simulink model "W06_city_highway_cs"  (R2019a)
settings: Solver=ode5  StartTime=0.0  StopTime=inf  FixedStep=1/60  RelTol=1e-3
PreLoadFcn:
  | mbxruntime.callbacks.PreLoadFcn(bdroot);
PostLoadFcn:
  | mbxruntime.callbacks.PostLoadFcn(bdroot);
InitFcn:
  | mbxruntime.callbacks.InitFcn(bdroot);
StartFcn:
  | mbxruntime.callbacks.StartFcn(bdroot);
StopFcn:
  | mbxruntime.callbacks.StopFcn(bdroot);
model workspace: external: MAT-File .\W06_city_highway_cs_hws.mat (data not in the file)
undefined symbols (not defined in the file or in its folder): DiscIntNeverNeededParam, FovAzimuth, FovAzimuthDefined, FovElevation, FovElevationDefined, Header, InitImageOutputDir, LocationX, LocationXDefined, LocationY, LocationYDefined, LocationZ, LocationZDefined, Orientation, OrientationPitch, OrientationPitchDefined, OrientationRoll, OrientationRollDefined, OrientationYaw, OrientationYawDefined, Poses, Poses_SL_Info, Position, W06_city_highway_cs_0270c22595f3b0e3, W06_city_highway_cs_086892688dd32ddc, W06_city_highway_cs_328c49ac39fca66b, W06_city_highway_cs_35ce05381b8ebe8c, W06_city_highway_cs_47b384f162638175, W06_city_highway_cs_766f76ce4de94dd5, W06_city_highway_cs_8c547f67cb81ffba, W06_city_highway_cs_aed52f2a7724a4f9, W06_city_highway_cs_Audi_A8_Sedan_1_Path_pathUniqueID, W06_city_highway_cs_b74cbb1f9f7331b5, W06_city_highway_cs_Citroen_C3_Hatchback_1_Path_pathUniqueID, W06_city_highway_cs_d395f8835e0c28b3, W06_city_highway_cs_e5f9d1759e19e2b4, W06_city_highway_cs_Toyota_Previa_MPV_1_Path_pathUniqueID
libraries: adeye_lib x26, simulink_extras x24, robotlib x7, sharedtransform x4, PreScanSimulinkLibrary x2, PreScanUsefulBlocks x1
(part 5 of 8)

== system W06_city_highway_cs/BMW_X5_SUV_2/HumViewCamera_CM_Demux ==
  In1 : Inport
  Selector : Selector  NumberOfDimensions=2  InputPortWidth=3  IndexOptions=Index vector (dialog),Index vector (dialog)  Indices=-1,1:hres  OutputSizes=1,1
  Selector1 : Selector  NumberOfDimensions=2  InputPortWidth=3  IndexOptions=Index vector (dialog),Index vector (dialog)  Indices=-1,hres+1:hres*2  OutputSizes=1,1
  Selector2 : Selector  NumberOfDimensions=2  InputPortWidth=3  IndexOptions=Index vector (dialog),Index vector (dialog)  Indices=-1,hres*2+1:hres*3  OutputSizes=1,1
  R : Outport
  G : Outport  Port=2
  B : Outport  Port=3
  wires:
  In1/1 -> Selector1/1, Selector/1, Selector2/1
  Selector/1 -> R/1
  Selector1/1 -> G/1
  Selector2/1 -> B/1

== system W06_city_highway_cs/BMW_X5_SUV_2/Mux_Camera_1_TA ==
  Location : Inport  Tag=inport/Camera_TA  OutDataTypeStr=double  PortDimensions=3  BusOutputAsStruct=on
  Orientation : Inport  Tag=inport/Camera_TA  Port=2  OutDataTypeStr=double  PortDimensions=3  BusOutputAsStruct=on
  IntensityFactorRGBMono : Inport  Tag=inport/Camera_TA  Port=3  OutDataTypeStr=double  PortDimensions=3  BusOutputAsStruct=on
  FoVAzimuth : Inport  Tag=inport/Camera_TA  Port=4  OutDataTypeStr=double  PortDimensions=1  BusOutputAsStruct=on
  FoVElevation : Inport  Tag=inport/Camera_TA  Port=5  OutDataTypeStr=double  PortDimensions=1  BusOutputAsStruct=on
  MisAlignMountPos : Inport  Tag=inport/Camera_TA  Port=6  OutDataTypeStr=double  PortDimensions=3  BusOutputAsStruct=on
  MisAlignMountOrient : Inport  Tag=inport/Camera_TA  Port=7  OutDataTypeStr=double  PortDimensions=3  BusOutputAsStruct=on
  Bus Assignment TA : BusAssignment  AssignedSignals=LocationX,LocationY,LocationZ,OrientationRoll,OrientationPitch,OrientationYaw,IntensityFactorR,IntensityFactorG,IntensityFactorB,FoVAzimuth,FoVElevation,MisalignMountPosX,MisalignMountPosY,MisalignMountPosZ,MisalignMountOrientX,MisalignMountOrientY,MisalignMountOrientZ,LocationXDefined,LocationYDefined,LocationZDefined,OrientationRollDefined,OrientationPitchDefined,OrientationYawDefined,IntensityFactorRDefined,IntensityFactorGDefined,IntensityFactorBDefined,FoVAzimuthDefined,FoVElevationDefined,MisalignMountPosXDefined,MisalignMountPosYDefined,MisalignMountPosZDefined,MisalignMountOrientXDefined,MisalignMountOrientYDefined,MisalignMountOrientZDefined
  ENABLE : Constant  Tag=ENABLE  Value=true
  IntensityFactorRGBMono_vec : Demux  Outputs=3
  Location_vec : Demux  Outputs=3
  MisAlignMountOrient_vec : Demux  Outputs=3
  MisAlignMountPos_vec : Demux  Outputs=3
  Orientation_vec : Demux  Outputs=3
  TA_bus : Subsystem
  TA : Outport  Tag=outport/Camera_TA/CameraSensor  OutDataTypeStr=Bus: PRESCAN_CAMERASENSOR_TA  PortDimensions=1  SampleTime=1/60
  wires:
  Bus Assignment TA/1 -> TA/1
  Location/1 -> Location_vec/1
  Location_vec/1 -> Bus Assignment TA/2
  Location_vec/2 -> Bus Assignment TA/3
  Location_vec/3 -> Bus Assignment TA/4
  Orientation/1 -> Orientation_vec/1
  Orientation_vec/1 -> Bus Assignment TA/5
  Orientation_vec/2 -> Bus Assignment TA/6
  Orientation_vec/3 -> Bus Assignment TA/7
  IntensityFactorRGBMono/1 -> IntensityFactorRGBMono_vec/1
  IntensityFactorRGBMono_vec/1 -> Bus Assignment TA/8
  IntensityFactorRGBMono_vec/2 -> Bus Assignment TA/9
  IntensityFactorRGBMono_vec/3 -> Bus Assignment TA/10
  FoVAzimuth/1 -> Bus Assignment TA/11
  FoVElevation/1 -> Bus Assignment TA/12
  MisAlignMountPos/1 -> MisAlignMountPos_vec/1
  MisAlignMountPos_vec/1 -> Bus Assignment TA/13
  MisAlignMountPos_vec/2 -> Bus Assignment TA/14
  MisAlignMountPos_vec/3 -> Bus Assignment TA/15
  MisAlignMountOrient/1 -> MisAlignMountOrient_vec/1
  MisAlignMountOrient_vec/1 -> Bus Assignment TA/16
  MisAlignMountOrient_vec/2 -> Bus Assignment TA/17
  MisAlignMountOrient_vec/3 -> Bus Assignment TA/18
  ENABLE/1 -> Bus Assignment TA/19, Bus Assignment TA/20, Bus Assignment TA/21, Bus Assignment TA/22, Bus Assignment TA/23, Bus Assignment TA/24, Bus Assignment TA/25, Bus Assignment TA/26, Bus Assignment TA/27, Bus Assignment TA/28, Bus Assignment TA/29, Bus Assignment TA/30, Bus Assignment TA/31, Bus Assignment TA/32, Bus Assignment TA/33, Bus Assignment TA/34, Bus Assignment TA/35
  TA_bus/1(bus) -> Bus Assignment TA/1

== system W06_city_highway_cs/BMW_X5_SUV_2/Mux_Camera_2_TA ==
  Location : Inport  Tag=inport/Camera_TA  OutDataTypeStr=double  PortDimensions=3  BusOutputAsStruct=on
  Orientation : Inport  Tag=inport/Camera_TA  Port=2  OutDataTypeStr=double  PortDimensions=3  BusOutputAsStruct=on
  IntensityFactorRGBMono : Inport  Tag=inport/Camera_TA  Port=3  OutDataTypeStr=double  PortDimensions=3  BusOutputAsStruct=on
  FoVAzimuth : Inport  Tag=inport/Camera_TA  Port=4  OutDataTypeStr=double  PortDimensions=1  BusOutputAsStruct=on
  FoVElevation : Inport  Tag=inport/Camera_TA  Port=5  OutDataTypeStr=double  PortDimensions=1  BusOutputAsStruct=on
  MisAlignMountPos : Inport  Tag=inport/Camera_TA  Port=6  OutDataTypeStr=double  PortDimensions=3  BusOutputAsStruct=on
  MisAlignMountOrient : Inport  Tag=inport/Camera_TA  Port=7  OutDataTypeStr=double  PortDimensions=3  BusOutputAsStruct=on
  Bus Assignment TA : BusAssignment  AssignedSignals=LocationX,LocationY,LocationZ,OrientationRoll,OrientationPitch,OrientationYaw,IntensityFactorR,IntensityFactorG,IntensityFactorB,FoVAzimuth,FoVElevation,MisalignMountPosX,MisalignMountPosY,MisalignMountPosZ,MisalignMountOrientX,MisalignMountOrientY,MisalignMountOrientZ,LocationXDefined,LocationYDefined,LocationZDefined,OrientationRollDefined,OrientationPitchDefined,OrientationYawDefined,IntensityFactorRDefined,IntensityFactorGDefined,IntensityFactorBDefined,FoVAzimuthDefined,FoVElevationDefined,MisalignMountPosXDefined,MisalignMountPosYDefined,MisalignMountPosZDefined,MisalignMountOrientXDefined,MisalignMountOrientYDefined,MisalignMountOrientZDefined
  ENABLE : Constant  Tag=ENABLE  Value=true
  IntensityFactorRGBMono_vec : Demux  Outputs=3
  Location_vec : Demux  Outputs=3
  MisAlignMountOrient_vec : Demux  Outputs=3
  MisAlignMountPos_vec : Demux  Outputs=3
  Orientation_vec : Demux  Outputs=3
  TA_bus : Subsystem
  TA : Outport  Tag=outport/Camera_TA/CameraSensor  OutDataTypeStr=Bus: PRESCAN_CAMERASENSOR_TA  PortDimensions=1  SampleTime=1/60
  wires:
  Bus Assignment TA/1 -> TA/1
  Location/1 -> Location_vec/1
  Location_vec/1 -> Bus Assignment TA/2
  Location_vec/2 -> Bus Assignment TA/3
  Location_vec/3 -> Bus Assignment TA/4
  Orientation/1 -> Orientation_vec/1
  Orientation_vec/1 -> Bus Assignment TA/5
  Orientation_vec/2 -> Bus Assignment TA/6
  Orientation_vec/3 -> Bus Assignment TA/7
  IntensityFactorRGBMono/1 -> IntensityFactorRGBMono_vec/1
  IntensityFactorRGBMono_vec/1 -> Bus Assignment TA/8
  IntensityFactorRGBMono_vec/2 -> Bus Assignment TA/9
  IntensityFactorRGBMono_vec/3 -> Bus Assignment TA/10
  FoVAzimuth/1 -> Bus Assignment TA/11
  FoVElevation/1 -> Bus Assignment TA/12
  MisAlignMountPos/1 -> MisAlignMountPos_vec/1
  MisAlignMountPos_vec/1 -> Bus Assignment TA/13
  MisAlignMountPos_vec/2 -> Bus Assignment TA/14
  MisAlignMountPos_vec/3 -> Bus Assignment TA/15
  MisAlignMountOrient/1 -> MisAlignMountOrient_vec/1
  MisAlignMountOrient_vec/1 -> Bus Assignment TA/16
  MisAlignMountOrient_vec/2 -> Bus Assignment TA/17
  MisAlignMountOrient_vec/3 -> Bus Assignment TA/18
  ENABLE/1 -> Bus Assignment TA/19, Bus Assignment TA/20, Bus Assignment TA/21, Bus Assignment TA/22, Bus Assignment TA/23, Bus Assignment TA/24, Bus Assignment TA/25, Bus Assignment TA/26, Bus Assignment TA/27, Bus Assignment TA/28, Bus Assignment TA/29, Bus Assignment TA/30, Bus Assignment TA/31, Bus Assignment TA/32, Bus Assignment TA/33, Bus Assignment TA/34, Bus Assignment TA/35
  TA_bus/1(bus) -> Bus Assignment TA/1

== system W06_city_highway_cs/BMW_X5_SUV_2/Mux_Camera_tl_TA ==
  Location : Inport  Tag=inport/Camera_TA  OutDataTypeStr=double  PortDimensions=3  BusOutputAsStruct=on
  Orientation : Inport  Tag=inport/Camera_TA  Port=2  OutDataTypeStr=double  PortDimensions=3  BusOutputAsStruct=on
  IntensityFactorRGBMono : Inport  Tag=inport/Camera_TA  Port=3  OutDataTypeStr=double  PortDimensions=3  BusOutputAsStruct=on
  FoVAzimuth : Inport  Tag=inport/Camera_TA  Port=4  OutDataTypeStr=double  PortDimensions=1  BusOutputAsStruct=on
  FoVElevation : Inport  Tag=inport/Camera_TA  Port=5  OutDataTypeStr=double  PortDimensions=1  BusOutputAsStruct=on
  MisAlignMountPos : Inport  Tag=inport/Camera_TA  Port=6  OutDataTypeStr=double  PortDimensions=3  BusOutputAsStruct=on
  MisAlignMountOrient : Inport  Tag=inport/Camera_TA  Port=7  OutDataTypeStr=double  PortDimensions=3  BusOutputAsStruct=on
  Bus Assignment TA : BusAssignment  AssignedSignals=LocationX,LocationY,LocationZ,OrientationRoll,OrientationPitch,OrientationYaw,IntensityFactorR,IntensityFactorG,IntensityFactorB,FoVAzimuth,FoVElevation,MisalignMountPosX,MisalignMountPosY,MisalignMountPosZ,MisalignMountOrientX,MisalignMountOrientY,MisalignMountOrientZ,LocationXDefined,LocationYDefined,LocationZDefined,OrientationRollDefined,OrientationPitchDefined,OrientationYawDefined,IntensityFactorRDefined,IntensityFactorGDefined,IntensityFactorBDefined,FoVAzimuthDefined,FoVElevationDefined,MisalignMountPosXDefined,MisalignMountPosYDefined,MisalignMountPosZDefined,MisalignMountOrientXDefined,MisalignMountOrientYDefined,MisalignMountOrientZDefined
  ENABLE : Constant  Tag=ENABLE  Value=true
  IntensityFactorRGBMono_vec : Demux  Outputs=3
  Location_vec : Demux  Outputs=3
  MisAlignMountOrient_vec : Demux  Outputs=3
  MisAlignMountPos_vec : Demux  Outputs=3
  Orientation_vec : Demux  Outputs=3
  TA_bus : Subsystem
  TA : Outport  Tag=outport/Camera_TA/CameraSensor  OutDataTypeStr=Bus: PRESCAN_CAMERASENSOR_TA  PortDimensions=1  SampleTime=1/60
  wires:
  Bus Assignment TA/1 -> TA/1
  Location/1 -> Location_vec/1
  Location_vec/1 -> Bus Assignment TA/2
  Location_vec/2 -> Bus Assignment TA/3
  Location_vec/3 -> Bus Assignment TA/4
  Orientation/1 -> Orientation_vec/1
  Orientation_vec/1 -> Bus Assignment TA/5
  Orientation_vec/2 -> Bus Assignment TA/6
  Orientation_vec/3 -> Bus Assignment TA/7
  IntensityFactorRGBMono/1 -> IntensityFactorRGBMono_vec/1
  IntensityFactorRGBMono_vec/1 -> Bus Assignment TA/8
  IntensityFactorRGBMono_vec/2 -> Bus Assignment TA/9
  IntensityFactorRGBMono_vec/3 -> Bus Assignment TA/10
  FoVAzimuth/1 -> Bus Assignment TA/11
  FoVElevation/1 -> Bus Assignment TA/12
  MisAlignMountPos/1 -> MisAlignMountPos_vec/1
  MisAlignMountPos_vec/1 -> Bus Assignment TA/13
  MisAlignMountPos_vec/2 -> Bus Assignment TA/14
  MisAlignMountPos_vec/3 -> Bus Assignment TA/15
  MisAlignMountOrient/1 -> MisAlignMountOrient_vec/1
  MisAlignMountOrient_vec/1 -> Bus Assignment TA/16
  MisAlignMountOrient_vec/2 -> Bus Assignment TA/17
  MisAlignMountOrient_vec/3 -> Bus Assignment TA/18
  ENABLE/1 -> Bus Assignment TA/19, Bus Assignment TA/20, Bus Assignment TA/21, Bus Assignment TA/22, Bus Assignment TA/23, Bus Assignment TA/24, Bus Assignment TA/25, Bus Assignment TA/26, Bus Assignment TA/27, Bus Assignment TA/28, Bus Assignment TA/29, Bus Assignment TA/30, Bus Assignment TA/31, Bus Assignment TA/32, Bus Assignment TA/33, Bus Assignment TA/34, Bus Assignment TA/35
  TA_bus/1(bus) -> Bus Assignment TA/1

== system W06_city_highway_cs/BMW_X5_SUV_2/Mux_HumViewCamera_TA ==
  Location : Inport  Tag=inport/Camera_TA  OutDataTypeStr=double  PortDimensions=3  BusOutputAsStruct=on
  Orientation : Inport  Tag=inport/Camera_TA  Port=2  OutDataTypeStr=double  PortDimensions=3  BusOutputAsStruct=on
  IntensityFactorRGBMono : Inport  Tag=inport/Camera_TA  Port=3  OutDataTypeStr=double  PortDimensions=3  BusOutputAsStruct=on
  FoVAzimuth : Inport  Tag=inport/Camera_TA  Port=4  OutDataTypeStr=double  PortDimensions=1  BusOutputAsStruct=on
  FoVElevation : Inport  Tag=inport/Camera_TA  Port=5  OutDataTypeStr=double  PortDimensions=1  BusOutputAsStruct=on
  MisAlignMountPos : Inport  Tag=inport/Camera_TA  Port=6  OutDataTypeStr=double  PortDimensions=3  BusOutputAsStruct=on
  MisAlignMountOrient : Inport  Tag=inport/Camera_TA  Port=7  OutDataTypeStr=double  PortDimensions=3  BusOutputAsStruct=on
  Bus Assignment TA : BusAssignment  AssignedSignals=LocationX,LocationY,LocationZ,OrientationRoll,OrientationPitch,OrientationYaw,IntensityFactorR,IntensityFactorG,IntensityFactorB,FoVAzimuth,FoVElevation,MisalignMountPosX,MisalignMountPosY,MisalignMountPosZ,MisalignMountOrientX,MisalignMountOrientY,MisalignMountOrientZ,LocationXDefined,LocationYDefined,LocationZDefined,OrientationRollDefined,OrientationPitchDefined,OrientationYawDefined,IntensityFactorRDefined,IntensityFactorGDefined,IntensityFactorBDefined,FoVAzimuthDefined,FoVElevationDefined,MisalignMountPosXDefined,MisalignMountPosYDefined,MisalignMountPosZDefined,MisalignMountOrientXDefined,MisalignMountOrientYDefined,MisalignMountOrientZDefined
  ENABLE : Constant  Tag=ENABLE  Value=true
  IntensityFactorRGBMono_vec : Demux  Outputs=3
  Location_vec : Demux  Outputs=3
  MisAlignMountOrient_vec : Demux  Outputs=3
  MisAlignMountPos_vec : Demux  Outputs=3
  Orientation_vec : Demux  Outputs=3
  TA_bus : Subsystem
  TA : Outport  Tag=outport/Camera_TA/CameraSensor  OutDataTypeStr=Bus: PRESCAN_CAMERASENSOR_TA  PortDimensions=1  SampleTime=1/60
  wires:
  Bus Assignment TA/1 -> TA/1
  Location/1 -> Location_vec/1
  Location_vec/1 -> Bus Assignment TA/2
  Location_vec/2 -> Bus Assignment TA/3
  Location_vec/3 -> Bus Assignment TA/4
  Orientation/1 -> Orientation_vec/1
  Orientation_vec/1 -> Bus Assignment TA/5
  Orientation_vec/2 -> Bus Assignment TA/6
  Orientation_vec/3 -> Bus Assignment TA/7
  IntensityFactorRGBMono/1 -> IntensityFactorRGBMono_vec/1
  IntensityFactorRGBMono_vec/1 -> Bus Assignment TA/8
  IntensityFactorRGBMono_vec/2 -> Bus Assignment TA/9
  IntensityFactorRGBMono_vec/3 -> Bus Assignment TA/10
  FoVAzimuth/1 -> Bus Assignment TA/11
  FoVElevation/1 -> Bus Assignment TA/12
  MisAlignMountPos/1 -> MisAlignMountPos_vec/1
  MisAlignMountPos_vec/1 -> Bus Assignment TA/13
  MisAlignMountPos_vec/2 -> Bus Assignment TA/14
  MisAlignMountPos_vec/3 -> Bus Assignment TA/15
  MisAlignMountOrient/1 -> MisAlignMountOrient_vec/1
  MisAlignMountOrient_vec/1 -> Bus Assignment TA/16
  MisAlignMountOrient_vec/2 -> Bus Assignment TA/17
  MisAlignMountOrient_vec/3 -> Bus Assignment TA/18
  ENABLE/1 -> Bus Assignment TA/19, Bus Assignment TA/20, Bus Assignment TA/21, Bus Assignment TA/22, Bus Assignment TA/23, Bus Assignment TA/24, Bus Assignment TA/25, Bus Assignment TA/26, Bus Assignment TA/27, Bus Assignment TA/28, Bus Assignment TA/29, Bus Assignment TA/30, Bus Assignment TA/31, Bus Assignment TA/32, Bus Assignment TA/33, Bus Assignment TA/34, Bus Assignment TA/35
  TA_bus/1(bus) -> Bus Assignment TA/1

== system W06_city_highway_cs/BMW_X5_SUV_2/Mux_PointCloudSensor_1_TA ==
  Location : Inport  Tag=inport/PointCloud_TA  OutDataTypeStr=double  PortDimensions=3  BusOutputAsStruct=on
  Orientation : Inport  Tag=inport/PointCloud_TA  Port=2  OutDataTypeStr=double  PortDimensions=3  BusOutputAsStruct=on
  FovAzimuth : Inport  Tag=inport/PointCloud_TA  Port=3  OutDataTypeStr=double  PortDimensions=1  BusOutputAsStruct=on
  FovElevation : Inport  Tag=inport/PointCloud_TA  Port=4  OutDataTypeStr=double  PortDimensions=1  BusOutputAsStruct=on
  Bus Assignment TA : BusAssignment  AssignedSignals=LocationX,LocationY,LocationZ,OrientationRoll,OrientationPitch,OrientationYaw,FovAzimuth,FovElevation,LocationXDefined,LocationYDefined,LocationZDefined,OrientationRollDefined,OrientationPitchDefined,OrientationYawDefined,FovAzimuthDefined,FovElevationDefined
  ENABLE : Constant  Tag=ENABLE  Value=true
  Location_vec : Demux  Outputs=3
  Orientation_vec : Demux  Outputs=3
  TA_bus : Subsystem
  TA : Outport  Tag=outport/SensorTA  OutDataTypeStr=Bus: PRESCAN_PCS_TA_DATA  PortDimensions=1  SampleTime=1/60
  wires:
  Bus Assignment TA/1 -> TA/1
  Location/1 -> Location_vec/1
  Location_vec/1 -> Bus Assignment TA/2
  Location_vec/2 -> Bus Assignment TA/3
  Location_vec/3 -> Bus Assignment TA/4
  Orientation/1 -> Orientation_vec/1
  Orientation_vec/1 -> Bus Assignment TA/5
  Orientation_vec/2 -> Bus Assignment TA/6
  Orientation_vec/3 -> Bus Assignment TA/7
  FovAzimuth/1 -> Bus Assignment TA/8
  FovElevation/1 -> Bus Assignment TA/9
  ENABLE/1 -> Bus Assignment TA/10, Bus Assignment TA/11, Bus Assignment TA/12, Bus Assignment TA/13, Bus Assignment TA/14, Bus Assignment TA/15, Bus Assignment TA/16, Bus Assignment TA/17
  TA_bus/1(bus) -> Bus Assignment TA/1

== system W06_city_highway_cs/BMW_X5_SUV_2/Mux_PointCloudSensor_2_TA ==
  Location : Inport  Tag=inport/PointCloud_TA  OutDataTypeStr=double  PortDimensions=3  BusOutputAsStruct=on
  Orientation : Inport  Tag=inport/PointCloud_TA  Port=2  OutDataTypeStr=double  PortDimensions=3  BusOutputAsStruct=on
  FovAzimuth : Inport  Tag=inport/PointCloud_TA  Port=3  OutDataTypeStr=double  PortDimensions=1  BusOutputAsStruct=on
  FovElevation : Inport  Tag=inport/PointCloud_TA  Port=4  OutDataTypeStr=double  PortDimensions=1  BusOutputAsStruct=on
  Bus Assignment TA : BusAssignment  AssignedSignals=LocationX,LocationY,LocationZ,OrientationRoll,OrientationPitch,OrientationYaw,FovAzimuth,FovElevation,LocationXDefined,LocationYDefined,LocationZDefined,OrientationRollDefined,OrientationPitchDefined,OrientationYawDefined,FovAzimuthDefined,FovElevationDefined
  ENABLE : Constant  Tag=ENABLE  Value=true
  Location_vec : Demux  Outputs=3
  Orientation_vec : Demux  Outputs=3
  TA_bus : Subsystem
  TA : Outport  Tag=outport/SensorTA  OutDataTypeStr=Bus: PRESCAN_PCS_TA_DATA  PortDimensions=1  SampleTime=1/60
  wires:
  Bus Assignment TA/1 -> TA/1
  Location/1 -> Location_vec/1
  Location_vec/1 -> Bus Assignment TA/2
  Location_vec/2 -> Bus Assignment TA/3
  Location_vec/3 -> Bus Assignment TA/4
  Orientation/1 -> Orientation_vec/1
  Orientation_vec/1 -> Bus Assignment TA/5
  Orientation_vec/2 -> Bus Assignment TA/6
  Orientation_vec/3 -> Bus Assignment TA/7
  FovAzimuth/1 -> Bus Assignment TA/8
  FovElevation/1 -> Bus Assignment TA/9
  ENABLE/1 -> Bus Assignment TA/10, Bus Assignment TA/11, Bus Assignment TA/12, Bus Assignment TA/13, Bus Assignment TA/14, Bus Assignment TA/15, Bus Assignment TA/16, Bus Assignment TA/17
  TA_bus/1(bus) -> Bus Assignment TA/1

== system W06_city_highway_cs/BMW_X5_SUV_2/Mux_PointCloudSensor_3_TA ==
  Location : Inport  Tag=inport/PointCloud_TA  OutDataTypeStr=double  PortDimensions=3  BusOutputAsStruct=on
  Orientation : Inport  Tag=inport/PointCloud_TA  Port=2  OutDataTypeStr=double  PortDimensions=3  BusOutputAsStruct=on
  FovAzimuth : Inport  Tag=inport/PointCloud_TA  Port=3  OutDataTypeStr=double  PortDimensions=1  BusOutputAsStruct=on
  FovElevation : Inport  Tag=inport/PointCloud_TA  Port=4  OutDataTypeStr=double  PortDimensions=1  BusOutputAsStruct=on
  Bus Assignment TA : BusAssignment  AssignedSignals=LocationX,LocationY,LocationZ,OrientationRoll,OrientationPitch,OrientationYaw,FovAzimuth,FovElevation,LocationXDefined,LocationYDefined,LocationZDefined,OrientationRollDefined,OrientationPitchDefined,OrientationYawDefined,FovAzimuthDefined,FovElevationDefined
  ENABLE : Constant  Tag=ENABLE  Value=true
  Location_vec : Demux  Outputs=3
  Orientation_vec : Demux  Outputs=3
  TA_bus : Subsystem
  TA : Outport  Tag=outport/SensorTA  OutDataTypeStr=Bus: PRESCAN_PCS_TA_DATA  PortDimensions=1  SampleTime=1/60
  wires:
  Bus Assignment TA/1 -> TA/1
  Location/1 -> Location_vec/1
  Location_vec/1 -> Bus Assignment TA/2
  Location_vec/2 -> Bus Assignment TA/3
  Location_vec/3 -> Bus Assignment TA/4
  Orientation/1 -> Orientation_vec/1
  Orientation_vec/1 -> Bus Assignment TA/5
  Orientation_vec/2 -> Bus Assignment TA/6
  Orientation_vec/3 -> Bus Assignment TA/7
  FovAzimuth/1 -> Bus Assignment TA/8
  FovElevation/1 -> Bus Assignment TA/9
  ENABLE/1 -> Bus Assignment TA/10, Bus Assignment TA/11, Bus Assignment TA/12, Bus Assignment TA/13, Bus Assignment TA/14, Bus Assignment TA/15, Bus Assignment TA/16, Bus Assignment TA/17
  TA_bus/1(bus) -> Bus Assignment TA/1

== system W06_city_highway_cs/BMW_X5_SUV_2/Mux_PointCloudSensor_4_TA ==
  Location : Inport  Tag=inport/PointCloud_TA  OutDataTypeStr=double  PortDimensions=3  BusOutputAsStruct=on
  Orientation : Inport  Tag=inport/PointCloud_TA  Port=2  OutDataTypeStr=double  PortDimensions=3  BusOutputAsStruct=on
  FovAzimuth : Inport  Tag=inport/PointCloud_TA  Port=3  OutDataTypeStr=double  PortDimensions=1  BusOutputAsStruct=on
  FovElevation : Inport  Tag=inport/PointCloud_TA  Port=4  OutDataTypeStr=double  PortDimensions=1  BusOutputAsStruct=on
  Bus Assignment TA : BusAssignment  AssignedSignals=LocationX,LocationY,LocationZ,OrientationRoll,OrientationPitch,OrientationYaw,FovAzimuth,FovElevation,LocationXDefined,LocationYDefined,LocationZDefined,OrientationRollDefined,OrientationPitchDefined,OrientationYawDefined,FovAzimuthDefined,FovElevationDefined
  ENABLE : Constant  Tag=ENABLE  Value=true
  Location_vec : Demux  Outputs=3
  Orientation_vec : Demux  Outputs=3
  TA_bus : Subsystem
  TA : Outport  Tag=outport/SensorTA  OutDataTypeStr=Bus: PRESCAN_PCS_TA_DATA  PortDimensions=1  SampleTime=1/60
  wires:
  Bus Assignment TA/1 -> TA/1
  Location/1 -> Location_vec/1
  Location_vec/1 -> Bus Assignment TA/2
  Location_vec/2 -> Bus Assignment TA/3
  Location_vec/3 -> Bus Assignment TA/4
  Orientation/1 -> Orientation_vec/1
  Orientation_vec/1 -> Bus Assignment TA/5
  Orientation_vec/2 -> Bus Assignment TA/6
  Orientation_vec/3 -> Bus Assignment TA/7
  FovAzimuth/1 -> Bus Assignment TA/8
  FovElevation/1 -> Bus Assignment TA/9
  ENABLE/1 -> Bus Assignment TA/10, Bus Assignment TA/11, Bus Assignment TA/12, Bus Assignment TA/13, Bus Assignment TA/14, Bus Assignment TA/15, Bus Assignment TA/16, Bus Assignment TA/17
  TA_bus/1(bus) -> Bus Assignment TA/1

== system W06_city_highway_cs/BMW_X5_SUV_2/Mux_Radar_1_TA ==
  Location : Inport  Tag=inport/Radar_TA  OutDataTypeStr=double  PortDimensions=3  BusOutputAsStruct=on
  Orientation : Inport  Tag=inport/Radar_TA  Port=2  OutDataTypeStr=double  PortDimensions=3  BusOutputAsStruct=on
  Range : Inport  Tag=inport/Radar_TA  Port=3  OutDataTypeStr=double  PortDimensions=1  BusOutputAsStruct=on
  NoiseAzimuthIllumination : Inport  Tag=inport/Radar_TA  Port=4  OutDataTypeStr=double  PortDimensions=1  BusOutputAsStruct=on
  NoiseAziIlluType : Inport  Tag=inport/Radar_TA  Port=5  OutDataTypeStr=uint32  PortDimensions=1  BusOutputAsStruct=on
  NoiseElevationIllumination : Inport  Tag=inport/Radar_TA  Port=6  OutDataTypeStr=double  PortDimensions=1  BusOutputAsStruct=on
  NoiseElevIlluType : Inport  Tag=inport/Radar_TA  Port=7  OutDataTypeStr=uint32  PortDimensions=1  BusOutputAsStruct=on
  NoiseAzimuthReflection : Inport  Tag=inport/Radar_TA  Port=8  OutDataTypeStr=double  PortDimensions=1  BusOutputAsStruct=on
  NoiseAziReflectType : Inport  Tag=inport/Radar_TA  Port=9  OutDataTypeStr=uint32  PortDimensions=1  BusOutputAsStruct=on
  NoiseElevationReflection : Inport  Tag=inport/Radar_TA  Port=10  OutDataTypeStr=double  PortDimensions=1  BusOutputAsStruct=on
  NoiseElevReflectType : Inport  Tag=inport/Radar_TA  Port=11  OutDataTypeStr=uint32  PortDimensions=1  BusOutputAsStruct=on
  NoiseRange : Inport  Tag=inport/Radar_TA  Port=12  OutDataTypeStr=double  PortDimensions=1  BusOutputAsStruct=on
  NoiseRangeType : Inport  Tag=inport/Radar_TA  Port=13  OutDataTypeStr=uint32  PortDimensions=1  BusOutputAsStruct=on
  Bus Assignment TA : BusAssignment  AssignedSignals=LocationX,LocationY,LocationZ,OrientationRoll,OrientationPitch,OrientationYaw,Range,NoiseAzimuthIllumination,NoiseAziIlluType,NoiseElevationIllumination,NoiseElevIlluType,NoiseAzimuthReflection,NoiseAziReflectType,NoiseElevationReflection,NoiseElevReflectType,NoiseRange,NoiseRangeType,LocationXDefined,LocationYDefined,LocationZDefined,OrientationRollDefined,OrientationPitchDefined,OrientationYawDefined,RangeDefined,NoiseAzimuthIlluminationDefined,NoiseAziIlluTypeDefined,NoiseElevationIlluminationDefined,NoiseElevIlluTypeDefined,NoiseAzimuthReflectionDefined,NoiseAziReflectTypeDefined,NoiseElevationReflectionDefined,NoiseElevReflectTypeDefined,NoiseRangeDefined,NoiseRangeTypeDefined
  ENABLE : Constant  Tag=ENABLE  Value=true
  Location_vec : Demux  Outputs=3
  Orientation_vec : Demux  Outputs=3
  TA_bus : Subsystem
  TA : Outport  Tag=outport/Radar_TA  OutDataTypeStr=Bus: PRESCAN_SCANNERSENSOR_TA  PortDimensions=1  SampleTime=1/60
  wires:
  Bus Assignment TA/1 -> TA/1
  Location/1 -> Location_vec/1
  Location_vec/1 -> Bus Assignment TA/2
  Location_vec/2 -> Bus Assignment TA/3
  Location_vec/3 -> Bus Assignment TA/4
  Orientation/1 -> Orientation_vec/1
  Orientation_vec/1 -> Bus Assignment TA/5
  Orientation_vec/2 -> Bus Assignment TA/6
  Orientation_vec/3 -> Bus Assignment TA/7
  Range/1 -> Bus Assignment TA/8
  NoiseAzimuthIllumination/1 -> Bus Assignment TA/9
  NoiseAziIlluType/1 -> Bus Assignment TA/10
  NoiseElevationIllumination/1 -> Bus Assignment TA/11
  NoiseElevIlluType/1 -> Bus Assignment TA/12
  NoiseAzimuthReflection/1 -> Bus Assignment TA/13
  NoiseAziReflectType/1 -> Bus Assignment TA/14
  NoiseElevationReflection/1 -> Bus Assignment TA/15
  NoiseElevReflectType/1 -> Bus Assignment TA/16
  NoiseRange/1 -> Bus Assignment TA/17
  NoiseRangeType/1 -> Bus Assignment TA/18
  ENABLE/1 -> Bus Assignment TA/19, Bus Assignment TA/20, Bus Assignment TA/21, Bus Assignment TA/22, Bus Assignment TA/23, Bus Assignment TA/24, Bus Assignment TA/25, Bus Assignment TA/26, Bus Assignment TA/27, Bus Assignment TA/28, Bus Assignment TA/29, Bus Assignment TA/30, Bus Assignment TA/31, Bus Assignment TA/32, Bus Assignment TA/33, Bus Assignment TA/34, Bus Assignment TA/35
  TA_bus/1(bus) -> Bus Assignment TA/1

== system W06_city_highway_cs/BMW_X5_SUV_2/PointCloudSensor_1_Angles_Demux ==
  In2 : Inport
  Selector : Selector  NumberOfDimensions=2  InputPortWidth=3  IndexOptions=Index vector (dialog),Index vector (dialog)  Indices=-1,offset+1:(offset+hres)  OutputSizes=1,1
  Selector1 : Selector  NumberOfDimensions=2  InputPortWidth=3  IndexOptions=Index vector (dialog),Index vector (dialog)  Indices=-1,(offset+hres+1):(offset+2*hres)  OutputSizes=1,1
  Theta : Outport
  Phi : Outport  Port=2
  wires:
  Selector1/1 -> Phi/1
  Selector/1 -> Theta/1
  In2/1 -> Selector/1, Selector1/1

== system W06_city_highway_cs/BMW_X5_SUV_2/PointCloudSensor_1_Intensity_Demux ==
  In1 : Inport
  Selector3 : Selector  NumberOfDimensions=2  InputPortWidth=3  IndexOptions=Index vector (dialog),Index vector (dialog)  Indices=-1,offset+1:(offset+hres)  OutputSizes=1,1
  Intensity : Outport
  wires:
  Selector3/1 -> Intensity/1
  In1/1 -> Selector3/1

== system W06_city_highway_cs/BMW_X5_SUV_2/PointCloudSensor_1_Range_Demux ==
  In1 : Inport
  Selector : Selector  NumberOfDimensions=2  InputPortWidth=3  IndexOptions=Index vector (dialog),Index vector (dialog)  Indices=-1,offset+1:(offset+hres)  OutputSizes=1,1
  Range : Outport
  wires:
  Selector/1 -> Range/1
  In1/1 -> Selector/1

== system W06_city_highway_cs/BMW_X5_SUV_2/PointCloudSensor_2_Angles_Demux ==
  In2 : Inport
  Selector : Selector  NumberOfDimensions=2  InputPortWidth=3  IndexOptions=Index vector (dialog),Index vector (dialog)  Indices=-1,offset+1:(offset+hres)  OutputSizes=1,1
  Selector1 : Selector  NumberOfDimensions=2  InputPortWidth=3  IndexOptions=Index vector (dialog),Index vector (dialog)  Indices=-1,(offset+hres+1):(offset+2*hres)  OutputSizes=1,1
  Theta : Outport
  Phi : Outport  Port=2
  wires:
  Selector1/1 -> Phi/1
  Selector/1 -> Theta/1
  In2/1 -> Selector/1, Selector1/1

== system W06_city_highway_cs/BMW_X5_SUV_2/PointCloudSensor_2_Intensity_Demux ==
  In1 : Inport
  Selector3 : Selector  NumberOfDimensions=2  InputPortWidth=3  IndexOptions=Index vector (dialog),Index vector (dialog)  Indices=-1,offset+1:(offset+hres)  OutputSizes=1,1
  Intensity : Outport
  wires:
  Selector3/1 -> Intensity/1
  In1/1 -> Selector3/1

== system W06_city_highway_cs/BMW_X5_SUV_2/PointCloudSensor_2_Range_Demux ==
  In1 : Inport
  Selector : Selector  NumberOfDimensions=2  InputPortWidth=3  IndexOptions=Index vector (dialog),Index vector (dialog)  Indices=-1,offset+1:(offset+hres)  OutputSizes=1,1
  Range : Outport
  wires:
  Selector/1 -> Range/1
  In1/1 -> Selector/1

== system W06_city_highway_cs/BMW_X5_SUV_2/PointCloudSensor_3_Angles_Demux ==
  In2 : Inport
  Selector : Selector  NumberOfDimensions=2  InputPortWidth=3  IndexOptions=Index vector (dialog),Index vector (dialog)  Indices=-1,offset+1:(offset+hres)  OutputSizes=1,1
  Selector1 : Selector  NumberOfDimensions=2  InputPortWidth=3  IndexOptions=Index vector (dialog),Index vector (dialog)  Indices=-1,(offset+hres+1):(offset+2*hres)  OutputSizes=1,1
  Theta : Outport
  Phi : Outport  Port=2
  wires:
  Selector1/1 -> Phi/1
  Selector/1 -> Theta/1
  In2/1 -> Selector/1, Selector1/1

== system W06_city_highway_cs/BMW_X5_SUV_2/PointCloudSensor_3_Intensity_Demux ==
  In1 : Inport
  Selector3 : Selector  NumberOfDimensions=2  InputPortWidth=3  IndexOptions=Index vector (dialog),Index vector (dialog)  Indices=-1,offset+1:(offset+hres)  OutputSizes=1,1
  Intensity : Outport
  wires:
  Selector3/1 -> Intensity/1
  In1/1 -> Selector3/1

== system W06_city_highway_cs/BMW_X5_SUV_2/PointCloudSensor_3_Range_Demux ==
  In1 : Inport
  Selector : Selector  NumberOfDimensions=2  InputPortWidth=3  IndexOptions=Index vector (dialog),Index vector (dialog)  Indices=-1,offset+1:(offset+hres)  OutputSizes=1,1
  Range : Outport
  wires:
  Selector/1 -> Range/1
  In1/1 -> Selector/1

== system W06_city_highway_cs/BMW_X5_SUV_2/PointCloudSensor_4_Angles_Demux ==
  In2 : Inport
  Selector : Selector  NumberOfDimensions=2  InputPortWidth=3  IndexOptions=Index vector (dialog),Index vector (dialog)  Indices=-1,offset+1:(offset+hres)  OutputSizes=1,1
  Selector1 : Selector  NumberOfDimensions=2  InputPortWidth=3  IndexOptions=Index vector (dialog),Index vector (dialog)  Indices=-1,(offset+hres+1):(offset+2*hres)  OutputSizes=1,1
  Theta : Outport
  Phi : Outport  Port=2
  wires:
  Selector1/1 -> Phi/1
  Selector/1 -> Theta/1
  In2/1 -> Selector/1, Selector1/1

== system W06_city_highway_cs/BMW_X5_SUV_2/PointCloudSensor_4_Intensity_Demux ==
  In1 : Inport
  Selector3 : Selector  NumberOfDimensions=2  InputPortWidth=3  IndexOptions=Index vector (dialog),Index vector (dialog)  Indices=-1,offset+1:(offset+hres)  OutputSizes=1,1
  Intensity : Outport
  wires:
  Selector3/1 -> Intensity/1
  In1/1 -> Selector3/1

== system W06_city_highway_cs/BMW_X5_SUV_2/PointCloudSensor_4_Range_Demux ==
  In1 : Inport
  Selector : Selector  NumberOfDimensions=2  InputPortWidth=3  IndexOptions=Index vector (dialog),Index vector (dialog)  Indices=-1,offset+1:(offset+hres)  OutputSizes=1,1
  Range : Outport
  wires:
  Selector/1 -> Range/1
  In1/1 -> Selector/1

== system W06_city_highway_cs/BMW_X5_SUV_2/Radar_1_Demux ==
  Radar : Inport
  Bus Selector1 : BusSelector  OutputSignals=ActiveBeamID[-],Range[m],DopplerVelocity[ms-1],DopplerVelocityX[ms-1],DopplerVelocityY[ms-1],DopplerVelocityZ[ms-1],Theta[deg],Phi[deg],TargetID[-],TargetTypeID[-],EnergyLoss[dB],Alpha[deg],Beta[deg]  OutputAsBus=on
  ScannerSensorLegacyBusConversion : PreScanUsefulBlocks/ScannerSensorLegacyBusConversion  MAXMESSAGES=MAXMESSAGES
  Radar Data : Outport
  wires:
  Bus Selector1/1 -> Radar Data/1
  ScannerSensorLegacyBusConversion/1 -> Bus Selector1/1
  Radar/1 -> ScannerSensorLegacyBusConversion/1

== system W06_city_highway_cs/BMW_X5_SUV_2/SELF_Demux ==
  SELF : Inport  OutDataTypeStr=Bus: PRESCAN_SELFSENSORDATA
  Bus Selector : BusSelector  OutputSignals=PositionX,PositionY,PositionZ,OrientationRoll,OrientationPitch,OrientationYaw,Velocity,Yaw_rate,Lat,Long,Alt
  Demux2 : Demux  Outputs=3
  Gain : Gain  Gain=180/pi
  Gain1 : Gain  Gain=180/pi
  Vector Concatenate1 : Concatenate  NumInputs=3
  compas converter : Subsystem
  x [m] : Outport
  y [m] : Outport  Port=2
  z [m] : Outport  Port=3
  rotx [deg] : Outport  Port=4
  roty [deg] : Outport  Port=5
  rotz [deg] : Outport  Port=6
  GPS lat [deg] : Outport  Port=7
  GPS long [deg] : Outport  Port=8
  GPS alt [m] : Outport  Port=9
  velocity [m/s] : Outport  Port=10
  heading [deg] : Outport  Port=11
  yaw rate [deg/s] : Outport  Port=12
  wires:
  Bus Selector/11 -> GPS alt [m]/1  "<Alt>"
  Bus Selector/10 -> GPS long [deg]/1  "<Long>"
  Bus Selector/9 -> GPS lat [deg]/1  "<Lat>"
  Bus Selector/8 -> Gain1/1  "<Yaw_rate>"
  Bus Selector/7 -> velocity [m/s]/1  "<Velocity>"
  Bus Selector/6 -> compas converter/1(rotz [rad]), Vector Concatenate1/3  "<OrientationYaw>"
  Bus Selector/5 -> Vector Concatenate1/2  "<OrientationPitch>"
  Bus Selector/4 -> Vector Concatenate1/1  "<OrientationRoll>"
  Vector Concatenate1/1 -> Gain/1
  Bus Selector/3 -> z [m]/1  "<PositionZ>"
  Bus Selector/2 -> y [m]/1  "<PositionY>"
  Bus Selector/1 -> x [m]/1  "<PositionX>"
  SELF/1 -> Bus Selector/1
  Gain/1 -> Demux2/1
  Demux2/1 -> rotx [deg]/1
  Demux2/2 -> roty [deg]/1
  Demux2/3 -> rotz [deg]/1
  compas converter/1(heading [deg]) -> heading [deg]/1
  Gain1/1 -> yaw rate [deg/s]/1

== system W06_city_highway_cs/Citroen_C3_Hatchback_1/Car_Pos_and_Orient ==
  In1 : Inport
  In2 : Inport  Port=2
  In3 : Inport  Port=3
  In4 : Inport  Port=4
  In5 : Inport  Port=5
  In6 : Inport  Port=6
  Data Type Conversion : DataTypeConversion
  Data Type Conversion1 : DataTypeConversion
  Data Type Conversion2 : DataTypeConversion
  Degrees to Radians1 : simulink_extras/Transformations/Degrees to Radians
  Degrees to Radians2 : simulink_extras/Transformations/Degrees to Radians
  Degrees to Radians5 : simulink_extras/Transformations/Degrees to Radians
  Mux : Mux
  Rotation Angles to Quaternions : sharedtransform/Rotation Angles to Quaternions  rotationOrder=XYZ  aMode=aMode
      settings: SourceProductName=Aerospace Blockset  SourceProductBaseCode=AE
  Vector Concatenate2 : Concatenate  NumInputs=3
  Out1 : Outport
  wires:
  Degrees to Radians1/1 -> Vector Concatenate2/2
  Degrees to Radians5/1 -> Vector Concatenate2/1
  Vector Concatenate2/1 -> Rotation Angles to Quaternions/1
  Degrees to Radians2/1 -> Vector Concatenate2/3
  In1/1 -> Data Type Conversion/1
  In2/1 -> Data Type Conversion1/1
  In3/1 -> Data Type Conversion2/1
  In4/1 -> Degrees to Radians5/1
  In5/1 -> Degrees to Radians1/1
  In6/1 -> Degrees to Radians2/1
  Data Type Conversion/1 -> Mux/1
  Data Type Conversion1/1 -> Mux/2
  Data Type Conversion2/1 -> Mux/3
  Rotation Angles to Quaternions/1 -> Mux/4
  Mux/1 -> Out1/1

== system W06_city_highway_cs/Citroen_C3_Hatchback_1/SELF_Demux ==
  SELF : Inport  OutDataTypeStr=Bus: PRESCAN_SELFSENSORDATA
  Bus Selector : BusSelector  OutputSignals=PositionX,PositionY,PositionZ,OrientationRoll,OrientationPitch,OrientationYaw,Velocity,Yaw_rate,Lat,Long,Alt
  Demux2 : Demux  Outputs=3
  Gain : Gain  Gain=180/pi
  Gain1 : Gain  Gain=180/pi
  Vector Concatenate1 : Concatenate  NumInputs=3
  compas converter : Subsystem
  x [m] : Outport
  y [m] : Outport  Port=2
  z [m] : Outport  Port=3
  rotx [deg] : Outport  Port=4
  roty [deg] : Outport  Port=5
  rotz [deg] : Outport  Port=6
  GPS lat [deg] : Outport  Port=7
  GPS long [deg] : Outport  Port=8
  GPS alt [m] : Outport  Port=9
  velocity [m/s] : Outport  Port=10
  heading [deg] : Outport  Port=11
  yaw rate [deg/s] : Outport  Port=12
  wires:
  Bus Selector/11 -> GPS alt [m]/1  "<Alt>"
  Bus Selector/10 -> GPS long [deg]/1  "<Long>"
  Bus Selector/9 -> GPS lat [deg]/1  "<Lat>"
  Bus Selector/8 -> Gain1/1  "<Yaw_rate>"
  Bus Selector/7 -> velocity [m/s]/1  "<Velocity>"
  Bus Selector/6 -> compas converter/1(rotz [rad]), Vector Concatenate1/3  "<OrientationYaw>"
  Bus Selector/5 -> Vector Concatenate1/2  "<OrientationPitch>"
  Bus Selector/4 -> Vector Concatenate1/1  "<OrientationRoll>"
  Vector Concatenate1/1 -> Gain/1
  Bus Selector/3 -> z [m]/1  "<PositionZ>"
  Bus Selector/2 -> y [m]/1  "<PositionY>"
  Bus Selector/1 -> x [m]/1  "<PositionX>"
  SELF/1 -> Bus Selector/1
  Gain/1 -> Demux2/1
  Demux2/1 -> rotx [deg]/1
  Demux2/2 -> roty [deg]/1
  Demux2/3 -> rotz [deg]/1
  compas converter/1(heading [deg]) -> heading [deg]/1
  Gain1/1 -> yaw rate [deg/s]/1

== system W06_city_highway_cs/Citroen_C3_Hatchback_1/message_creator ==
  In1 : Inport
  Blank Message4 : robotlib/Blank Message  messageClass=Message  entityType=geometry_msgs/Pose  messageType=geometry_msgs/Pose  SampleTime=inf
      settings: SourceProductBaseCode=RO
  Bus Assignment3 : BusAssignment  AssignedSignals=Position.X,Position.Y,Position.Z,Orientation.W,Orientation.X,Orientation.Y,Orientation.Z
  Demux : Demux  Outputs=7
  Out1 : Outport
  wires:
  Blank Message4/1 -> Bus Assignment3/1
  Demux/4 -> Bus Assignment3/5
  Demux/3 -> Bus Assignment3/4
  Demux/5 -> Bus Assignment3/6
  Demux/7 -> Bus Assignment3/8
  Demux/2 -> Bus Assignment3/3
  In1/1 -> Demux/1
  Demux/6 -> Bus Assignment3/7
  Demux/1 -> Bus Assignment3/2
  Bus Assignment3/1 -> Out1/1

== system W06_city_highway_cs/MercedesBenz_Actros_2541_L_6x2_1/Car_Pos_and_Orient ==
  In1 : Inport
  In2 : Inport  Port=2
  In3 : Inport  Port=3
  In4 : Inport  Port=4
  In5 : Inport  Port=5
  In6 : Inport  Port=6
  Data Type Conversion : DataTypeConversion
  Data Type Conversion1 : DataTypeConversion
  Data Type Conversion2 : DataTypeConversion
  Degrees to Radians1 : simulink_extras/Transformations/Degrees to Radians
  Degrees to Radians2 : simulink_extras/Transformations/Degrees to Radians
  Degrees to Radians5 : simulink_extras/Transformations/Degrees to Radians
  Mux : Mux
  Rotation Angles to Quaternions : sharedtransform/Rotation Angles to Quaternions  rotationOrder=XYZ  aMode=aMode
      settings: SourceProductName=Aerospace Blockset  SourceProductBaseCode=AE
  Vector Concatenate2 : Concatenate  NumInputs=3
  Out1 : Outport
  wires:
  Degrees to Radians1/1 -> Vector Concatenate2/2
  Degrees to Radians5/1 -> Vector Concatenate2/1
  Vector Concatenate2/1 -> Rotation Angles to Quaternions/1
  Degrees to Radians2/1 -> Vector Concatenate2/3
  In1/1 -> Data Type Conversion/1
  In2/1 -> Data Type Conversion1/1
  In3/1 -> Data Type Conversion2/1
  In4/1 -> Degrees to Radians5/1
  In5/1 -> Degrees to Radians1/1
  In6/1 -> Degrees to Radians2/1
  Data Type Conversion/1 -> Mux/1
  Data Type Conversion1/1 -> Mux/2
  Data Type Conversion2/1 -> Mux/3
  Rotation Angles to Quaternions/1 -> Mux/4
  Mux/1 -> Out1/1

== system W06_city_highway_cs/MercedesBenz_Actros_2541_L_6x2_1/SELF_Demux ==
  SELF : Inport  OutDataTypeStr=Bus: PRESCAN_SELFSENSORDATA
  Bus Selector : BusSelector  OutputSignals=PositionX,PositionY,PositionZ,OrientationRoll,OrientationPitch,OrientationYaw,Velocity,Yaw_rate,Lat,Long,Alt
  Demux2 : Demux  Outputs=3
  Gain : Gain  Gain=180/pi
  Gain1 : Gain  Gain=180/pi
  Vector Concatenate1 : Concatenate  NumInputs=3
  compas converter : Subsystem
  x [m] : Outport
  y [m] : Outport  Port=2
  z [m] : Outport  Port=3
  rotx [deg] : Outport  Port=4
  roty [deg] : Outport  Port=5
  rotz [deg] : Outport  Port=6
  GPS lat [deg] : Outport  Port=7
  GPS long [deg] : Outport  Port=8
  GPS alt [m] : Outport  Port=9
  velocity [m/s] : Outport  Port=10
  heading [deg] : Outport  Port=11
  yaw rate [deg/s] : Outport  Port=12
  wires:
  Bus Selector/11 -> GPS alt [m]/1  "<Alt>"
  Bus Selector/10 -> GPS long [deg]/1  "<Long>"
  Bus Selector/9 -> GPS lat [deg]/1  "<Lat>"
  Bus Selector/8 -> Gain1/1  "<Yaw_rate>"
  Bus Selector/7 -> velocity [m/s]/1  "<Velocity>"
  Bus Selector/6 -> compas converter/1(rotz [rad]), Vector Concatenate1/3  "<OrientationYaw>"
  Bus Selector/5 -> Vector Concatenate1/2  "<OrientationPitch>"
  Bus Selector/4 -> Vector Concatenate1/1  "<OrientationRoll>"
  Vector Concatenate1/1 -> Gain/1
  Bus Selector/3 -> z [m]/1  "<PositionZ>"
  Bus Selector/2 -> y [m]/1  "<PositionY>"
  Bus Selector/1 -> x [m]/1  "<PositionX>"
  SELF/1 -> Bus Selector/1
  Gain/1 -> Demux2/1
  Demux2/1 -> rotx [deg]/1
  Demux2/2 -> roty [deg]/1
  Demux2/3 -> rotz [deg]/1
  compas converter/1(heading [deg]) -> heading [deg]/1
  Gain1/1 -> yaw rate [deg/s]/1

== system W06_city_highway_cs/MercedesBenz_Actros_2541_L_6x2_1/message_creator ==
  In1 : Inport
  Blank Message4 : robotlib/Blank Message  messageClass=Message  entityType=geometry_msgs/Pose  messageType=geometry_msgs/Pose  SampleTime=inf
      settings: SourceProductBaseCode=RO
  Bus Assignment3 : BusAssignment  AssignedSignals=Position.X,Position.Y,Position.Z,Orientation.W,Orientation.X,Orientation.Y,Orientation.Z
  Demux : Demux  Outputs=7
  Out1 : Outport
  wires:
  Blank Message4/1 -> Bus Assignment3/1
  Demux/4 -> Bus Assignment3/5
  Demux/3 -> Bus Assignment3/4
  Demux/5 -> Bus Assignment3/6
  Demux/7 -> Bus Assignment3/8
  Demux/2 -> Bus Assignment3/3
  In1/1 -> Demux/1
  Demux/6 -> Bus Assignment3/7
  Demux/1 -> Bus Assignment3/2
  Bus Assignment3/1 -> Out1/1

== system W06_city_highway_cs/RoadsideLight_NL_1/Green_Mux ==
  MSCD [Cd] : Inport
  Position (xyz) [m] : Inport  Port=2
  Orientation (RPY) [deg] : Inport  Port=3
  Color [-] : Inport  Port=4
  TextureResourceID [-] : Inport  Port=5
  Bus Creator : BusCreator  Inputs='Intensity','Position','Orientation','Color','TextureResourceID'  OutDataTypeStr=Bus: PRESCAN_VISULIGHTACTUATOR_DATA  NonVirtualBus=on
  Bus Creator1 : BusCreator  Inputs=3  OutDataTypeStr=Bus: PRESCAN_RGB_DATA  NonVirtualBus=on
  Bus Creator2 : BusCreator  Inputs=3  OutDataTypeStr=Bus: PRESCAN_RPY_DATA  NonVirtualBus=on
  Bus Creator3 : BusCreator  Inputs=3  OutDataTypeStr=Bus: PRESCAN_XYZ_DATA  NonVirtualBus=on
  Data Type Conversion : DataTypeConversion  OutDataTypeStr=int32  RndMeth=Nearest
  Degrees to Radians : simulink_extras/Transformations/Degrees to Radians
  Demux : Demux  Outputs=3
  Demux1 : Demux  Outputs=3
  Demux2 : Demux  Outputs=3
  Lights : Outport
  wires:
  TextureResourceID [-]/1 -> Data Type Conversion/1  "TextureResourceID"
  MSCD [Cd]/1 -> Bus Creator/1  "Intensity"
  Bus Creator/1 -> Lights/1
  Demux/1 -> Bus Creator1/1  "R"
  Demux/2 -> Bus Creator1/2  "G"
  Demux/3 -> Bus Creator1/3  "B"
  Color [-]/1 -> Demux/1  "Color"
  Bus Creator1/1 -> Bus Creator/4  "Color"
  Demux1/1 -> Bus Creator2/1  "Roll"
  Demux1/2 -> Bus Creator2/2  "Pitch"
  Demux1/3 -> Bus Creator2/3  "Yaw"
  Orientation (RPY) [deg]/1 -> Degrees to Radians/1  "Orientation"
  Bus Creator2/1 -> Bus Creator/3  "Orientation"
  Demux2/1 -> Bus Creator3/1  "X"
  Demux2/2 -> Bus Creator3/2  "Y"
  Demux2/3 -> Bus Creator3/3  "Z"
  Position (xyz) [m]/1 -> Demux2/1  "Position"
  Bus Creator3/1 -> Bus Creator/2  "Position"
  Data Type Conversion/1 -> Bus Creator/5  "TextureResourceID"
  Degrees to Radians/1 -> Demux1/1

== system W06_city_highway_cs/RoadsideLight_NL_1/Orange_Mux ==
  MSCD [Cd] : Inport
  Position (xyz) [m] : Inport  Port=2
  Orientation (RPY) [deg] : Inport  Port=3
  Color [-] : Inport  Port=4
  TextureResourceID [-] : Inport  Port=5
  Bus Creator : BusCreator  Inputs='Intensity','Position','Orientation','Color','TextureResourceID'  OutDataTypeStr=Bus: PRESCAN_VISULIGHTACTUATOR_DATA  NonVirtualBus=on
  Bus Creator1 : BusCreator  Inputs=3  OutDataTypeStr=Bus: PRESCAN_RGB_DATA  NonVirtualBus=on
  Bus Creator2 : BusCreator  Inputs=3  OutDataTypeStr=Bus: PRESCAN_RPY_DATA  NonVirtualBus=on
  Bus Creator3 : BusCreator  Inputs=3  OutDataTypeStr=Bus: PRESCAN_XYZ_DATA  NonVirtualBus=on
  Data Type Conversion : DataTypeConversion  OutDataTypeStr=int32  RndMeth=Nearest
  Degrees to Radians : simulink_extras/Transformations/Degrees to Radians
  Demux : Demux  Outputs=3
  Demux1 : Demux  Outputs=3
  Demux2 : Demux  Outputs=3
  Lights : Outport
  wires:
  TextureResourceID [-]/1 -> Data Type Conversion/1  "TextureResourceID"
  MSCD [Cd]/1 -> Bus Creator/1  "Intensity"
  Bus Creator/1 -> Lights/1
  Demux/1 -> Bus Creator1/1  "R"
  Demux/2 -> Bus Creator1/2  "G"
  Demux/3 -> Bus Creator1/3  "B"
  Color [-]/1 -> Demux/1  "Color"
  Bus Creator1/1 -> Bus Creator/4  "Color"
  Demux1/1 -> Bus Creator2/1  "Roll"
  Demux1/2 -> Bus Creator2/2  "Pitch"
  Demux1/3 -> Bus Creator2/3  "Yaw"
  Orientation (RPY) [deg]/1 -> Degrees to Radians/1  "Orientation"
  Bus Creator2/1 -> Bus Creator/3  "Orientation"
  Demux2/1 -> Bus Creator3/1  "X"
  Demux2/2 -> Bus Creator3/2  "Y"
  Demux2/3 -> Bus Creator3/3  "Z"
  Position (xyz) [m]/1 -> Demux2/1  "Position"
  Bus Creator3/1 -> Bus Creator/2  "Position"
  Data Type Conversion/1 -> Bus Creator/5  "TextureResourceID"
  Degrees to Radians/1 -> Demux1/1

== system W06_city_highway_cs/RoadsideLight_NL_1/Red_Mux ==
  MSCD [Cd] : Inport
  Position (xyz) [m] : Inport  Port=2
  Orientation (RPY) [deg] : Inport  Port=3
  Color [-] : Inport  Port=4
  TextureResourceID [-] : Inport  Port=5
  Bus Creator : BusCreator  Inputs='Intensity','Position','Orientation','Color','TextureResourceID'  OutDataTypeStr=Bus: PRESCAN_VISULIGHTACTUATOR_DATA  NonVirtualBus=on
  Bus Creator1 : BusCreator  Inputs=3  OutDataTypeStr=Bus: PRESCAN_RGB_DATA  NonVirtualBus=on
  Bus Creator2 : BusCreator  Inputs=3  OutDataTypeStr=Bus: PRESCAN_RPY_DATA  NonVirtualBus=on
  Bus Creator3 : BusCreator  Inputs=3  OutDataTypeStr=Bus: PRESCAN_XYZ_DATA  NonVirtualBus=on
  Data Type Conversion : DataTypeConversion  OutDataTypeStr=int32  RndMeth=Nearest
  Degrees to Radians : simulink_extras/Transformations/Degrees to Radians
  Demux : Demux  Outputs=3
  Demux1 : Demux  Outputs=3
  Demux2 : Demux  Outputs=3
  Lights : Outport
  wires:
  TextureResourceID [-]/1 -> Data Type Conversion/1  "TextureResourceID"
  MSCD [Cd]/1 -> Bus Creator/1  "Intensity"
  Bus Creator/1 -> Lights/1
  Demux/1 -> Bus Creator1/1  "R"
  Demux/2 -> Bus Creator1/2  "G"
  Demux/3 -> Bus Creator1/3  "B"
  Color [-]/1 -> Demux/1  "Color"
  Bus Creator1/1 -> Bus Creator/4  "Color"
  Demux1/1 -> Bus Creator2/1  "Roll"
  Demux1/2 -> Bus Creator2/2  "Pitch"
  Demux1/3 -> Bus Creator2/3  "Yaw"
  Orientation (RPY) [deg]/1 -> Degrees to Radians/1  "Orientation"
  Bus Creator2/1 -> Bus Creator/3  "Orientation"
  Demux2/1 -> Bus Creator3/1  "X"
  Demux2/2 -> Bus Creator3/2  "Y"
  Demux2/3 -> Bus Creator3/3  "Z"
  Position (xyz) [m]/1 -> Demux2/1  "Position"
  Bus Creator3/1 -> Bus Creator/2  "Position"
  Data Type Conversion/1 -> Bus Creator/5  "TextureResourceID"
  Degrees to Radians/1 -> Demux1/1

== system W06_city_highway_cs/RoadsideLight_NL_2/Green_Mux ==
  MSCD [Cd] : Inport
  Position (xyz) [m] : Inport  Port=2
  Orientation (RPY) [deg] : Inport  Port=3
  Color [-] : Inport  Port=4
  TextureResourceID [-] : Inport  Port=5
  Bus Creator : BusCreator  Inputs='Intensity','Position','Orientation','Color','TextureResourceID'  OutDataTypeStr=Bus: PRESCAN_VISULIGHTACTUATOR_DATA  NonVirtualBus=on
  Bus Creator1 : BusCreator  Inputs=3  OutDataTypeStr=Bus: PRESCAN_RGB_DATA  NonVirtualBus=on
  Bus Creator2 : BusCreator  Inputs=3  OutDataTypeStr=Bus: PRESCAN_RPY_DATA  NonVirtualBus=on
  Bus Creator3 : BusCreator  Inputs=3  OutDataTypeStr=Bus: PRESCAN_XYZ_DATA  NonVirtualBus=on
  Data Type Conversion : DataTypeConversion  OutDataTypeStr=int32  RndMeth=Nearest
  Degrees to Radians : simulink_extras/Transformations/Degrees to Radians
  Demux : Demux  Outputs=3
  Demux1 : Demux  Outputs=3
  Demux2 : Demux  Outputs=3
  Lights : Outport
  wires:
  TextureResourceID [-]/1 -> Data Type Conversion/1  "TextureResourceID"
  MSCD [Cd]/1 -> Bus Creator/1  "Intensity"
  Bus Creator/1 -> Lights/1
  Demux/1 -> Bus Creator1/1  "R"
  Demux/2 -> Bus Creator1/2  "G"
  Demux/3 -> Bus Creator1/3  "B"
  Color [-]/1 -> Demux/1  "Color"
  Bus Creator1/1 -> Bus Creator/4  "Color"
  Demux1/1 -> Bus Creator2/1  "Roll"
  Demux1/2 -> Bus Creator2/2  "Pitch"
  Demux1/3 -> Bus Creator2/3  "Yaw"
  Orientation (RPY) [deg]/1 -> Degrees to Radians/1  "Orientation"
  Bus Creator2/1 -> Bus Creator/3  "Orientation"
  Demux2/1 -> Bus Creator3/1  "X"
  Demux2/2 -> Bus Creator3/2  "Y"
  Demux2/3 -> Bus Creator3/3  "Z"
  Position (xyz) [m]/1 -> Demux2/1  "Position"
  Bus Creator3/1 -> Bus Creator/2  "Position"
  Data Type Conversion/1 -> Bus Creator/5  "TextureResourceID"
  Degrees to Radians/1 -> Demux1/1

== system W06_city_highway_cs/RoadsideLight_NL_2/Orange_Mux ==
  MSCD [Cd] : Inport
  Position (xyz) [m] : Inport  Port=2
  Orientation (RPY) [deg] : Inport  Port=3
  Color [-] : Inport  Port=4
  TextureResourceID [-] : Inport  Port=5
  Bus Creator : BusCreator  Inputs='Intensity','Position','Orientation','Color','TextureResourceID'  OutDataTypeStr=Bus: PRESCAN_VISULIGHTACTUATOR_DATA  NonVirtualBus=on
  Bus Creator1 : BusCreator  Inputs=3  OutDataTypeStr=Bus: PRESCAN_RGB_DATA  NonVirtualBus=on
  Bus Creator2 : BusCreator  Inputs=3  OutDataTypeStr=Bus: PRESCAN_RPY_DATA  NonVirtualBus=on
  Bus Creator3 : BusCreator  Inputs=3  OutDataTypeStr=Bus: PRESCAN_XYZ_DATA  NonVirtualBus=on
  Data Type Conversion : DataTypeConversion  OutDataTypeStr=int32  RndMeth=Nearest
  Degrees to Radians : simulink_extras/Transformations/Degrees to Radians
  Demux : Demux  Outputs=3
  Demux1 : Demux  Outputs=3
  Demux2 : Demux  Outputs=3
  Lights : Outport
  wires:
  TextureResourceID [-]/1 -> Data Type Conversion/1  "TextureResourceID"
  MSCD [Cd]/1 -> Bus Creator/1  "Intensity"
  Bus Creator/1 -> Lights/1
  Demux/1 -> Bus Creator1/1  "R"
  Demux/2 -> Bus Creator1/2  "G"
  Demux/3 -> Bus Creator1/3  "B"
  Color [-]/1 -> Demux/1  "Color"
  Bus Creator1/1 -> Bus Creator/4  "Color"
  Demux1/1 -> Bus Creator2/1  "Roll"
  Demux1/2 -> Bus Creator2/2  "Pitch"
  Demux1/3 -> Bus Creator2/3  "Yaw"
  Orientation (RPY) [deg]/1 -> Degrees to Radians/1  "Orientation"
  Bus Creator2/1 -> Bus Creator/3  "Orientation"
  Demux2/1 -> Bus Creator3/1  "X"
  Demux2/2 -> Bus Creator3/2  "Y"
  Demux2/3 -> Bus Creator3/3  "Z"
  Position (xyz) [m]/1 -> Demux2/1  "Position"
  Bus Creator3/1 -> Bus Creator/2  "Position"
  Data Type Conversion/1 -> Bus Creator/5  "TextureResourceID"
  Degrees to Radians/1 -> Demux1/1
